simulink model "FiniteGainOpAmp"  (R2024a)
settings: Solver=VariableStepAuto  StartTime=0.0  StopTime=0.002  MaxStep=0.00002  RelTol=1e-3  AbsTol=1e-3  EnableMultiTasking=on
libraries: fl_lib x12, nesl_utility x3
CloseFcn:
  | try,close(h1_FiniteGainOpAmp),end
  | clear h1_FiniteGainOpAmp
  | clear simlog_FiniteGainOpAmp
Description:
  | Finite-Gain Op-Amp
settings Model: Creator=The MathWorks, Inc.  LastModifiedBy=The MathWorks, Inc.
settings SolverCC: AutoScaleAbsTol=off  AlgebraicLoopSolver=TrustRegion
settings DataIOCC: LimitDataPoints=on  SaveFormat=Array  ReturnWorkspaceOutputs=off
settings OptimizationCC: LifeSpan=inf
settings DebuggingCC: SolverPrmCheckMsg=warning  UnconnectedInputMsg=warning  UnconnectedOutputMsg=warning  UnconnectedLineMsg=warning  AllowSymbolicDim=off  PregeneratedLibrarySubsystemCodeDiagnostic=none  SFUnexpectedBacktrackingDiag=warning  SFNoUnconditionalDefaultTransitionDiag=warning  SFExecutionAtInitializationDiag=none  ArithmeticOperatorsInVariantConditions=warning
settings HardwareCC: ProdBitPerPointer=32  ProdBitPerSizeT=32  ProdBitPerPtrDiffT=32  ProdLargestAtomicFloat=None  ProdIntDivRoundTo=Undefined  ProdEndianess=Unspecified  ProdWordSize=32  ProdHWDeviceType=32-bit Generic
settings ModelReferenceCC: EnableRefExpFcnMdlSchedulingChecks=on  PropagateSignalLabelsOutOfModel=off
settings SFSimCC: SimUseLocalCustomCode=off  CustomCodeUndefinedFunction=UseInterfaceOnly
settings RTWCC: RTWUseLocalCustomCode=off  GPUComputeCapability=3.5  DLArmComputeVersion=19.05
settings CodeAppCC: StateflowObjectComments=on
settings GRTTargetCC: TargetLangStandard=C89/C90 (ANSI)
settings ConfigComp: CovMetricSettings=dw  CovSaveCumulativeToWorkspaceVar=on  CovSaveSingleToWorkspaceVar=on  CovExternalEMLEnable=off  CovSFcnEnable=off
settings SimscapeCC: SimscapeLogType=all  SimscapeLogSimulationStatistics=on  SimscapeLogName=simlog_FiniteGainOpAmp  SimscapeLogDataHistory=10000

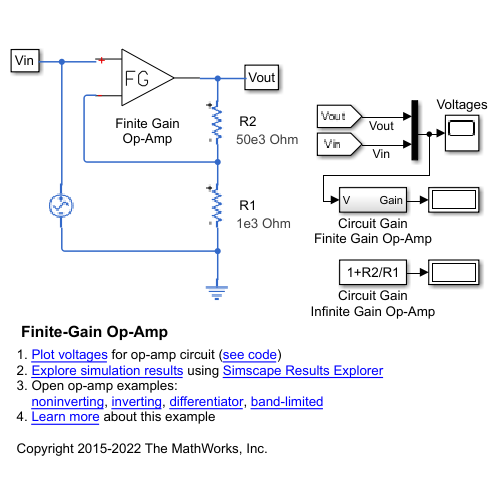
[thumbnail: Simulink's stored preview of the top-level diagram]
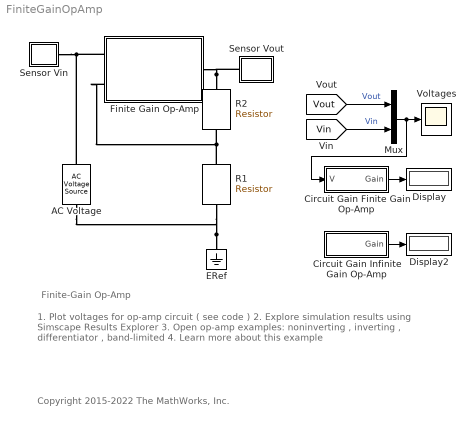
== system FiniteGainOpAmp ==
  note: 1. Plot voltages for op-amp circuit ( see code )
      | 2. Explore simulation results using Simscape Results Explorer
      | 3. Open op-amp examples:
      | noninverting , inverting , differentiator , band-limited
      | 4. Learn more about this example
  note: Finite-Gain Op-Amp
  note: Copyright 2015-2022 The MathWorks, Inc.
  AC Voltage : fl_lib/Electrical/Electrical Sources/AC Voltage Source  amp=0.1 V  shift=0 deg  frequency=1000 Hz
  Circuit Gain Finite Gain Op-Amp : Subsystem
  Circuit Gain Infinite Gain Op-Amp : Subsystem
      mask init:
      | set_param([gcb '/R1'],'Value',...
      |     get_param([bdroot '/R1'],'r'));
      | set_param([gcb '/R2'],'Value',...
      |     get_param([bdroot '/R2'],'r'));
      mask Display: disp('1+R2/R1')
  Display : Display
  Display2 : Display
  ERef : fl_lib/Electrical/Electrical Elements/Electrical Reference
  Finite Gain Op-Amp : Subsystem  Tag=PublishSubsystem
      mask Display:
      | % Plot Op-Amp
      | plot([1,2,1,1],[1,2,3,1])
      | 
      | % Band-limited symbol
      | % 'F'
      | plot([1.1,1.1],[1.7,2.2])
      | plot([1.1,1.27],[2.2,2.2])
      | plot([1.1,1.23],[2.2,2.2]-0.25)
      | 
      | % 'G'
      | plot([1.33,1.33],[2.1,1.8])
      | plot([1.33,1.4,1.45,1.5],[2.1,2.2,2.2,2.1])
      | plot([1.33,1.4,1.45,1.5,1.5,1.43],[1.8,1.7,1.7,1.8,1.9,1.9])
      | 
      | %  Connection
      | plot([2,2.5],[2,2])
      | plot([0.5, 1],[1.35 1.35])
      | plot([0.5, 1],[2.65 2.65])
      | 
      | % Scaling
      | color('white')
      | plot(0.5,0.8)
      | plot(2.5,3.2)
      | 
      | color('red')
      | port_label('LConn',1,'+');
      | port_label('LConn',2,'-');
  Mux : Mux  Inputs=2
  R1 : fl_lib/Electrical/Electrical Elements/Resistor  R=1e3 Ohm  i_specify=off  i_priority=High  i=0 A  i_nominal_specify=off  i_nominal_value=1  i_nominal_unit=A  v_specify=off  v_priority=High  v=0 V  v_nominal_specify=off  v_nominal_value=1  v_nominal_unit=V
      settings: AttributesFormatString=%<R> %<R_unit>
  R2 : fl_lib/Electrical/Electrical Elements/Resistor  R=50e3 Ohm  i_specify=off  i_priority=High  i=0 A  i_nominal_specify=off  i_nominal_value=1  i_nominal_unit=A  v_specify=off  v_priority=High  v=0 V  v_nominal_specify=off  v_nominal_value=1  v_nominal_unit=V
      settings: AttributesFormatString=%<R> %<R_unit>
  Sensor Vin : Subsystem
      mask Display: disp('Vin')
  Sensor Vout : Subsystem
      mask Display: disp('Vout')
  Voltages : Scope
  wires:
  Mux/1 -> Circuit Gain Finite Gain Op-Amp/1(V), Voltages/1
  [Vin] -> Mux/2  "Vin"
  [Vout] -> Mux/1  "Vout"
  Circuit Gain Infinite Gain Op-Amp/1(Gain) -> Display2/1
  Circuit Gain Finite Gain Op-Amp/1(Gain) -> Display/1
  connections:
  ERef/LConn1 -- AC Voltage/RConn1 -- R1/RConn1
  R2/LConn1 -- Sensor Vout/LConn1 -- Finite Gain Op-Amp/RConn1
  R2/RConn1 -- R1/LConn1 -- Finite Gain Op-Amp/LConn2
  Sensor Vin/LConn1 -- AC Voltage/LConn1 -- Finite Gain Op-Amp/LConn1

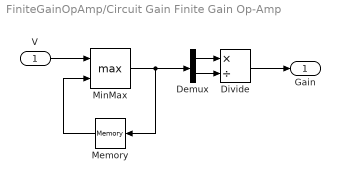
== system FiniteGainOpAmp/Circuit Gain Finite Gain Op-Amp ==
  V : Inport
  Demux : Demux  Outputs=2
  Divide : Product  Inputs=*/
  Memory : Memory  InitialCondition=1e-15  InheritSampleTime=on
  MinMax : MinMax  DisableCoverage=on  Function=max  Inputs=2  OutDataTypeStr=Inherit: Inherit via back propagation  ZeroCross=off
      settings: LockScale=on
  Gain : Outport  VectorParamsAs1DForOutWhenUnconnected=off
  wires:
  Divide/1 -> Gain/1
  Demux/2 -> Divide/2
  Memory/1 -> MinMax/2
  MinMax/1 -> Demux/1, Memory/1
  Demux/1 -> Divide/1
  V/1 -> MinMax/1

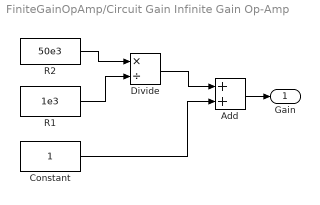
== system FiniteGainOpAmp/Circuit Gain Infinite Gain Op-Amp ==
  Add : Sum
  Constant : Constant
  Divide : Product  Inputs=*/
  R1 : Constant  Value=1e3
  R2 : Constant  Value=50e3
  Gain : Outport  VectorParamsAs1DForOutWhenUnconnected=off
  wires:
  R2/1 -> Divide/1
  R1/1 -> Divide/2
  Add/1 -> Gain/1
  Divide/1 -> Add/1
  Constant/1 -> Add/2

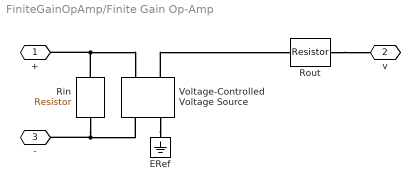
== system FiniteGainOpAmp/Finite Gain Op-Amp ==
  ERef : fl_lib/Electrical/Electrical Elements/Electrical Reference
  Rin : fl_lib/Electrical/Electrical Elements/Resistor  R=100e3 Ohm  i_specify=off  i_priority=High  i=0 A  i_nominal_specify=off  i_nominal_value=1  i_nominal_unit=A  v_specify=off  v_priority=High  v=0 V  v_nominal_specify=off  v_nominal_value=1  v_nominal_unit=V
  Rout : fl_lib/Electrical/Electrical Elements/Resistor  R=10 Ohm  i_specify=off  i_priority=High  i=0 A  i_nominal_specify=off  i_nominal_value=1  i_nominal_unit=A  v_specify=off  v_priority=High  v=0 V  v_nominal_specify=off  v_nominal_value=1  v_nominal_unit=V
  Voltage-Controlled Voltage Source : fl_lib/Electrical/Electrical Sources/Voltage-Controlled Voltage Source  K=1e5  v1_specify=off  v1_priority=High  v1=0 V  v1_nominal_specify=off  v1_nominal_value=1  v1_nominal_unit=V  v2_specify=off  v2_priority=High  v2=0 V  v2_nominal_specify=off  v2_nominal_value=1  v2_nominal_unit=V
      settings: InternalSimscapePortConfiguration="{\"Bottom\":[],\"Left\":[{\"id\":\"p1\",\"label\":\"+\",\"type\":\"foundation.electrical.electrical\"},{\"id\":\"p2\",\"label\":\"+\",\"type\":\"foundation.electrical.electrical\"}],\"Right\":[{\"id\":\"n1\",\"label\":\"-\",\"type\":\"foundation.electrical.electrical\"},{\"id\":\"n2\",\"label\":\"-\",\"type\":\"foundation.electrical.electrical\"}],\"Top\":[]}"
  + : PMIOPort  Side=Left
  v : PMIOPort  Port=2  Side=Right
  - : PMIOPort  Port=3  Side=Left
  connections:
  Rout/RConn1 -- v/RConn1
  Rin/LConn1 -- +/RConn1 -- Voltage-Controlled Voltage Source/LConn1
  Rin/RConn1 -- -/RConn1 -- Voltage-Controlled Voltage Source/RConn1
  Voltage-Controlled Voltage Source/LConn2 -- Rout/LConn1
  Voltage-Controlled Voltage Source/RConn2 -- ERef/LConn1

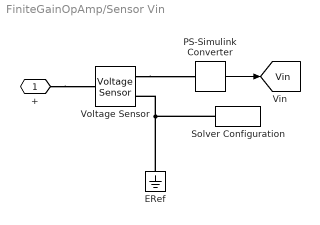
== system FiniteGainOpAmp/Sensor Vin ==
  ERef : fl_lib/Electrical/Electrical Elements/Electrical Reference
  PS-Simulink Converter : nesl_utility/PS-Simulink Converter  PhysicalDomain=network_engine_domain  SubClassName=ps_output  LeftPortType=input  RightPortType=output  PseudoPeriodic=off  Frequencies=[]  VectorFormat=1-D array  Unit=1  AffineConversion=off
  Solver Configuration : nesl_utility/Solver Configuration  PhysicalDomain=network_engine_domain  SubClassName=solver  LeftPortType=input  RightPortType=generic  Tones=[]  Harmonics=[]  SimulateNoise=off  Profile=off  UseLocalSampling=off  EnableSwitchedLinearOptims=on  FrequencyDomain=off  UseCCode=off  RelTol=0.001  AbsTol=1e-06  MinStep=1e-09  ToWorkspace=off  RevertToSquareIcSolve=off  NumHomotopyIterations=100  PhasorMode=off  PhasorModeNumHarmonics=1  ConsistencySolver=NEWTON_XTOL_AFTER_FTOL  IndexReductionMethod=DerivativeReplacement  DoDC=off  ResidualTolerance=1e-9  ConsistencyTolSource=GLOBAL  ConsistencyAbsTol=0.001  ConsistencyRelTol=0.001  ConsistencyTolFactor=0.001  UseLocalSolver=off  LocalSolverChoice=NE_BACKWARD_EULER_ADVANCER  ResolveIndetEquations=on  FunctionEvalNumThread=1  LocalSolverSampleTime=1e-6  DoFixedCost=off  MaxNonlinIter=3  MaxModeIter=2  ComputeImpulses=off  ImpulseIterations=2  LinearAlgebra=auto  LinearAlgebraNumThread=0  EquationFormulation=NE_TIME_EF  DelaysMemoryBudget=1024  AutomaticFiltering=on  FilteringTimeConstant=0.001  PartitionStorageMethod=AS_NEEDED  PartitionMemoryBudget=1024  PartitionMethod=FAST  MultibodyUseLocalSolver=off  MultibodyLocalSolverChoice=ODE1  MultibodyLocalSolverSampleTime=0.001
  Voltage Sensor : fl_lib/Electrical/Electrical Sensors/Voltage Sensor
  + : PMIOPort  Side=Left
  tag scope: Vin=global
  wires:
  PS-Simulink Converter/1 -> [Vin]
  connections:
  +/RConn1 -- Voltage Sensor/LConn1
  Voltage Sensor/RConn1 -- PS-Simulink Converter/LConn1
  ERef/LConn1 -- Solver Configuration/RConn1 -- Voltage Sensor/RConn2

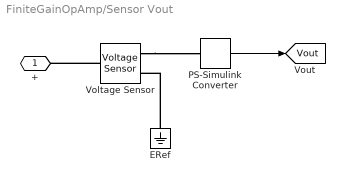
== system FiniteGainOpAmp/Sensor Vout ==
  ERef : fl_lib/Electrical/Electrical Elements/Electrical Reference
  PS-Simulink Converter : nesl_utility/PS-Simulink Converter  PhysicalDomain=network_engine_domain  SubClassName=ps_output  LeftPortType=input  RightPortType=output  PseudoPeriodic=off  Frequencies=[]  VectorFormat=1-D array  Unit=1  AffineConversion=off
  Voltage Sensor : fl_lib/Electrical/Electrical Sensors/Voltage Sensor
  + : PMIOPort  Side=Left
  tag scope: Vout=global
  wires:
  PS-Simulink Converter/1 -> [Vout]
  connections:
  ERef/LConn1 -- Voltage Sensor/RConn2
  Voltage Sensor/RConn1 -- PS-Simulink Converter/LConn1
  Voltage Sensor/LConn1 -- +/RConn1
